simulink model "Processing_sine_Wave"  (R2024b)
settings: Solver=FixedStepAuto  StartTime=0.0  StopTime=10.0  FixedStep=0.0001  RelTol=1e-3
settings Model: Creator=abdal  LastModifiedBy=abdal

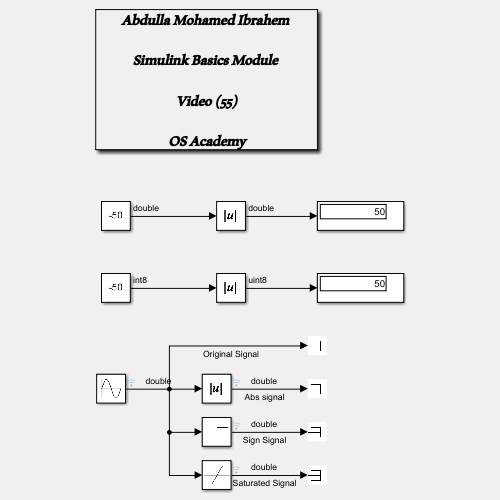
[thumbnail: Simulink's stored preview of the top-level diagram]
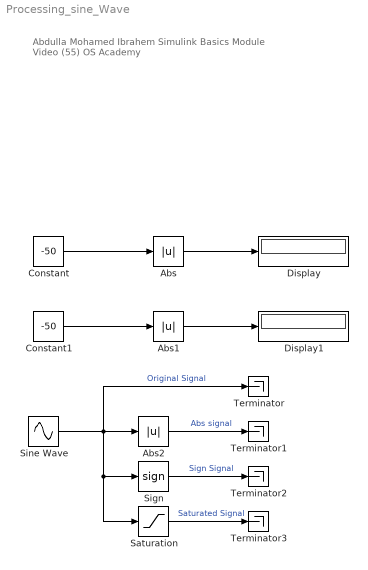
== system Processing_sine_Wave ==
  note: Abdulla Mohamed Ibrahem
      | Simulink Basics Module
      | Video (55)
      | OS Academy
  Abs : Abs  SaturateOnIntegerOverflow=off
  Abs1 : Abs  SaturateOnIntegerOverflow=off  OutDataTypeStr=Inherit: Inherit via internal rule
  Abs2 : Abs  SaturateOnIntegerOverflow=off
  Constant : Constant  Value=-50
  Constant1 : Constant  Value=-50  OutDataTypeStr=int8
  Display : Display
  Display1 : Display
  Saturation : Saturate
  Sign : Signum
  Sine Wave : Sin  SampleTime=0
  Terminator{,1..3} (4 alike) : Terminator
  wires:
  Constant/1 -> Abs/1
  Abs/1 -> Display/1
  Abs1/1 -> Display1/1
  Constant1/1 -> Abs1/1
  Sine Wave/1 -> Saturation/1, Sign/1, Terminator/1, Abs2/1  "Original Signal"
  Abs2/1 -> Terminator1/1  "Abs signal"
  Sign/1 -> Terminator2/1  "Sign Signal"
  Saturation/1 -> Terminator3/1  "Saturated Signal"
